simulink model "rlKinovaBallBalance_lags"  (R2024a)
settings: Solver=ode15s  StartTime=0.0  StopTime=inf  MaxStep=0.005  RelTol=1e-4  AbsTol=1e-4
values from neighbouring files (symbols this model uses):
  abs_max_torque_U = [6, 0.70, 2.12, 0.505]    [kinova_params.m]
  g = 3.71    [kinova_params.m]
  max_angular_vel = 2.0    (= 2)    [kinova_params.m]
  max_linear_vel = 0.6    [kinova_params.m]
  max_torque = [1.6; 0.6; 0.9; 0.5]    [kinova_params.m]
  max_torque_PD = [2.5; 0.6; 0.6; 0.3]    [kinova_params.m]
  R1_q0 = 0    [kinova_params.m]
  R2_q0 = deg2rad(20)    [kinova_params.m]
  R3_q0 = 0    [kinova_params.m]
  R4_q0 = deg2rad(135)    [kinova_params.m]
  R5_q0 = 0    [kinova_params.m]
  R6_q0 = deg2rad(-65)    [kinova_params.m]
  R7_q0 = deg2rad(-90)    [kinova_params.m]
  rlEpisodeFinalTime = 21    [kinova_params.m]
  rlStartTime = 0    [kinova_params.m]
  rlTimeStep = 0.01    [kinova_params.m]
  U0 = [-5.75, 0.10, -1.3, 0.0]    [kinova_params.m]
undefined symbols (not defined in the file or in its folder): Control, fluent0, L1, L2, L3, LS1, LS3, plate, R1, R2, R3, Rover, rover_path, RS1, RS3, Ts, vessel, X, Y, Z
libraries: sm_lib x251, nesl_utility x110, fl_lib x85, nesl_utility_internal x34, sdl_lib x20, simulink x16, ee_lib x10, mars_rover_lib x6, slpidlib x2, batteryecm_lib x2, robotalgslib x1, rllib x1
(part 3 of 13)

== system rlKinovaBallBalance_lags/Kinova Ball Balance/7 DOF Manipulator/Shoulder_Link ==
  Actuator1_AxisInvTransform : sm_lib/Frames and Transforms/Rigid Transform  RotationMethod=ArbitraryAxis  FollAlignAxisA=+X  BaseAlignAxisA=+Y  FollAlignAxisB=+Y  BaseAlignAxisB=+Z  RotationStandardAxis=+Z  RotationAngle=0  RotationAngleUnits=rad  RotationArbitraryAxis=[1, 0, 0]  RotationSequenceAxes=FollowerAxes  RotationSequence=XYX  RotationSequenceAngles=[0 0 0]  RotationSequenceAnglesUnits=deg  RotationMatrix=[1 0 0; 0 1 0; 0 0 1]  Quaternion=[1 0 0 0]  TranslationMethod=Cartesian  TranslationCartesianOffset=[0, 0, 0]  TranslationCartesianOffsetUnits=m  TranslationStandardAxis=+Z  TranslationStandardOffset=0  TranslationStandardOffsetUnits=m  TranslationROffset=0  TranslationROffsetUnits=m  TranslationThetaOffset=0  TranslationThetaOffsetUnits=deg  TranslationZOffset=0  TranslationZOffsetUnits=m
  Actuator2_AxisTransform : sm_lib/Frames and Transforms/Rigid Transform  RotationMethod=ArbitraryAxis  FollAlignAxisA=+X  BaseAlignAxisA=+Y  FollAlignAxisB=+Y  BaseAlignAxisB=+Z  RotationStandardAxis=+Z  RotationAngle=0  RotationAngleUnits=rad  RotationArbitraryAxis=[1, 0, 0]  RotationSequenceAxes=FollowerAxes  RotationSequence=XYX  RotationSequenceAngles=[0 0 0]  RotationSequenceAnglesUnits=deg  RotationMatrix=[1 0 0; 0 1 0; 0 0 1]  Quaternion=[1 0 0 0]  TranslationMethod=Cartesian  TranslationCartesianOffset=[0, 0, 0]  TranslationCartesianOffsetUnits=m  TranslationStandardAxis=+Z  TranslationStandardOffset=0  TranslationStandardOffsetUnits=m  TranslationROffset=0  TranslationROffsetUnits=m  TranslationThetaOffset=0  TranslationThetaOffsetUnits=deg  TranslationZOffset=0  TranslationZOffsetUnits=m
  Actuator2_OriginTransform : sm_lib/Frames and Transforms/Rigid Transform  RotationMethod=RotationSequence  FollAlignAxisA=+X  BaseAlignAxisA=+Y  FollAlignAxisB=+Y  BaseAlignAxisB=+Z  RotationStandardAxis=+Z  RotationAngle=0.0  RotationAngleUnits=deg  RotationArbitraryAxis=[0 0 1]  RotationSequenceAxes=BaseAxes  RotationSequence=XYZ  RotationSequenceAngles=[1.5708, 0, 0]  RotationSequenceAnglesUnits=rad  RotationMatrix=[1 0 0; 0 1 0; 0 0 1]  Quaternion=[1 0 0 0]  TranslationMethod=Cartesian  TranslationCartesianOffset=[0, 0.005375, -0.12838]  TranslationCartesianOffsetUnits=m  TranslationStandardAxis=+Z  TranslationStandardOffset=0  TranslationStandardOffsetUnits=m  TranslationROffset=0  TranslationROffsetUnits=m  TranslationThetaOffset=0  TranslationThetaOffsetUnits=deg  TranslationZOffset=0  TranslationZOffsetUnits=m
  Inertia : sm_lib/Body Elements/Inertia  InertiaType=Custom  Mass=2.009  MassUnits=kg  CenterOfMass=[0, 0, 0]  CenterOfMassUnits=m  MomentsOfInertia=[0.004508099999999999, 0.004769500000000001, 0.0013903]  MomentsOfInertiaUnits=kg*m^2  ProductsOfInertia=[-0.00045534, -1.8997e-06, -8.5826e-07]  ProductsOfInertiaUnits=kg*m^2  GraphicType=None  MarkerShape=Inertia  MarkerSize=20  GraphicVisPropType=SimpleVisualProperties  GraphicDiffuseColor=[0.5 0.5 0.5]  GraphicOpacity=1.0  GraphicSpecularColor=[0.5 0.5 0.5 1.0]  GraphicAmbientColor=[0.15 0.15 0.15 1.0]  GraphicEmissiveColor=[0.0 0.0 0.0 1.0]  GraphicShininess=75
  InertiaOriginTransform : sm_lib/Frames and Transforms/Rigid Transform  RotationMethod=RotationSequence  FollAlignAxisA=+X  BaseAlignAxisA=+Y  FollAlignAxisB=+Y  BaseAlignAxisB=+Z  RotationStandardAxis=+Z  RotationAngle=0.0  RotationAngleUnits=deg  RotationArbitraryAxis=[0 0 1]  RotationSequenceAxes=BaseAxes  RotationSequence=XYZ  RotationSequenceAngles=[0, 0, 0]  RotationSequenceAnglesUnits=rad  RotationMatrix=[1 0 0; 0 1 0; 0 0 1]  Quaternion=[1 0 0 0]  TranslationMethod=Cartesian  TranslationCartesianOffset=[-2.2888e-05, -0.010511, -0.075159]  TranslationCartesianOffsetUnits=m  TranslationStandardAxis=+Z  TranslationStandardOffset=0  TranslationStandardOffsetUnits=m  TranslationROffset=0  TranslationROffsetUnits=m  TranslationThetaOffset=0  TranslationThetaOffsetUnits=deg  TranslationZOffset=0  TranslationZOffsetUnits=m
  ReferenceFrame : sm_lib/Frames and Transforms/Reference Frame
  Shoulder Link : Subsystem  Variant=on  VariantControlMode=label  VariantControl=Choice  LabelModeActiveChoice=Choice_1
  VisualOriginTransform : sm_lib/Frames and Transforms/Rigid Transform  RotationMethod=RotationSequence  FollAlignAxisA=+X  BaseAlignAxisA=+Y  FollAlignAxisB=+Y  BaseAlignAxisB=+Z  RotationStandardAxis=+Z  RotationAngle=0.0  RotationAngleUnits=deg  RotationArbitraryAxis=[0 0 1]  RotationSequenceAxes=BaseAxes  RotationSequence=XYZ  RotationSequenceAngles=[0, 0, 0]  RotationSequenceAnglesUnits=rad  RotationMatrix=[1 0 0; 0 1 0; 0 0 1]  Quaternion=[1 0 0 0]  TranslationMethod=Cartesian  TranslationCartesianOffset=[0, 0, 0]  TranslationCartesianOffsetUnits=m  TranslationStandardAxis=+Z  TranslationStandardOffset=0  TranslationStandardOffsetUnits=m  TranslationROffset=0  TranslationROffsetUnits=m  TranslationThetaOffset=0  TranslationThetaOffsetUnits=deg  TranslationZOffset=0  TranslationZOffsetUnits=m
  F : PMIOPort  Side=Left
  F1 : PMIOPort  Port=2  Side=Right
  connections:
  Actuator1_AxisInvTransform/RConn1 -- F/RConn1
  Actuator2_AxisTransform/RConn1 -- F1/RConn1
  Actuator2_AxisTransform/LConn1 -- Actuator2_OriginTransform/RConn1
  Inertia/RConn1 -- InertiaOriginTransform/RConn1
  Actuator2_OriginTransform/LConn1 -- Actuator1_AxisInvTransform/LConn1 -- InertiaOriginTransform/LConn1 -- VisualOriginTransform/LConn1 -- ReferenceFrame/RConn1
  VisualOriginTransform/RConn1 -- Shoulder Link/RConn1

== system rlKinovaBallBalance_lags/Kinova Ball Balance/7 DOF Manipulator/Torque controller J2 ==
  q0 : Inport
  rl_t : Inport  Port=2
  Add Constant : Bias  Bias=U0(1)  SaturateOnIntegerOverflow=off
  Clock : Clock
  Compare To Constant : simulink/Logic and Bit Operations/Compare To Constant  relop=>=  const=rlStartTime  OutDataTypeStr=boolean
  Hold controller J2 : Subsystem
  Saturation : Saturate  UpperLimit=max_torque_PD(1)  LowerLimit=-max_torque_PD(1)
  Simulink-PS Converter1 : nesl_utility_internal/Simulink-PS Converter  PhysicalDomain=network_engine_domain  SubClassName=ps_input  LeftPortType=input  RightPortType=output  PseudoPeriodic=off  Frequencies=[]  NoiseDistribution=none  NoiseParameters=[]  Unit=1  AffineConversion=off  FilteringAndDerivatives=provide  SimscapeFilterOrder=1  InputFilterTimeConstant=0.001  UdotUserProvided=0
  Switch : Switch  Criteria=u2 > Threshold  ZeroCross=off  SaturateOnIntegerOverflow=off  InputSameDT=off
  Transfer Fcn : TransferFcn  Denominator=[0.01 1]
  q : PMIOPort  Side=Right
  w : PMIOPort  Port=2  Side=Right
  output : PMIOPort  Port=3  Side=Right
  torque J2 : Outport
  delta torque J2 : Outport  Port=2
  wires:
  rl_t/1 -> Switch/1
  Compare To Constant/1 -> Switch/2
  q0/1 -> Hold controller J2/1(q0)
  Clock/1 -> Compare To Constant/1
  Switch/1 -> Transfer Fcn/1
  Saturation/1 -> Add Constant/1
  Transfer Fcn/1 -> Simulink-PS Converter1/1
  Hold controller J2/1(hold t) -> delta torque J2/1, Saturation/1
  Add Constant/1 -> torque J2/1, Switch/3
  connections:
  Hold controller J2/LConn1 -- q/RConn1
  Hold controller J2/LConn2 -- w/RConn1
  output/RConn1 -- Simulink-PS Converter1/RConn1

== system rlKinovaBallBalance_lags/Kinova Ball Balance/7 DOF Manipulator/Torque controller J3 ==
  q0 : Inport
  rl_t : Inport  Port=2
  Add Constant : Bias  Bias=U0(2)  SaturateOnIntegerOverflow=off
  Clock : Clock
  Compare To Constant : simulink/Logic and Bit Operations/Compare To Constant  relop=>=  const=rlStartTime  OutDataTypeStr=boolean
  Hold controller J3 : Subsystem
  Saturation : Saturate  UpperLimit=max_torque_PD(2)  LowerLimit=-max_torque_PD(2)
  Simulink-PS Converter1 : nesl_utility_internal/Simulink-PS Converter  PhysicalDomain=network_engine_domain  SubClassName=ps_input  LeftPortType=input  RightPortType=output  PseudoPeriodic=off  Frequencies=[]  NoiseDistribution=none  NoiseParameters=[]  Unit=1  AffineConversion=off  FilteringAndDerivatives=provide  SimscapeFilterOrder=1  InputFilterTimeConstant=0.001  UdotUserProvided=0
  Switch : Switch  Criteria=u2 > Threshold  ZeroCross=off  SaturateOnIntegerOverflow=off  InputSameDT=off
  Transfer Fcn : TransferFcn  Denominator=[0.01 1]
  w : PMIOPort  Side=Right
  q : PMIOPort  Port=2  Side=Right
  output : PMIOPort  Port=3  Side=Right
  delta torque J3 : Outport
  torque J2 : Outport  Port=2
  wires:
  Hold controller J3/1(hold t) -> delta torque J3/1, Saturation/1
  Clock/1 -> Compare To Constant/1
  Switch/1 -> Transfer Fcn/1
  Compare To Constant/1 -> Switch/2
  q0/1 -> Hold controller J3/1(q0)
  Saturation/1 -> Add Constant/1
  rl_t/1 -> Switch/1
  Transfer Fcn/1 -> Simulink-PS Converter1/1
  Add Constant/1 -> Switch/3, torque J2/1
  connections:
  output/RConn1 -- Simulink-PS Converter1/RConn1
  Hold controller J3/LConn2 -- w/RConn1
  Hold controller J3/LConn1 -- q/RConn1

== system rlKinovaBallBalance_lags/Kinova Ball Balance/7 DOF Manipulator/Torque controller J6 ==
  q0 : Inport
  rl_t : Inport  Port=2
  Add Constant : Bias  Bias=U0(3)  SaturateOnIntegerOverflow=off
  Clock : Clock
  Compare To Constant : simulink/Logic and Bit Operations/Compare To Constant  relop=>=  const=rlStartTime  OutDataTypeStr=boolean
  Hold controller J6 : Subsystem
  Saturation : Saturate  UpperLimit=max_torque_PD(3)  LowerLimit=-max_torque_PD(3)
  Simulink-PS Converter1 : nesl_utility_internal/Simulink-PS Converter  PhysicalDomain=network_engine_domain  SubClassName=ps_input  LeftPortType=input  RightPortType=output  PseudoPeriodic=off  Frequencies=[]  NoiseDistribution=none  NoiseParameters=[]  Unit=1  AffineConversion=off  FilteringAndDerivatives=provide  SimscapeFilterOrder=1  InputFilterTimeConstant=0.001  UdotUserProvided=0
  Switch : Switch  Criteria=u2 > Threshold  ZeroCross=off  SaturateOnIntegerOverflow=off  InputSameDT=off
  Transfer Fcn : TransferFcn  Denominator=[0.01 1]
  q : PMIOPort  Side=Right
  output : PMIOPort  Port=2  Side=Right
  w : PMIOPort  Port=3  Side=Right
  delta torque J6 : Outport
  torque J6 : Outport  Port=2
  wires:
  Hold controller J6/1(hold t) -> delta torque J6/1, Saturation/1
  Clock/1 -> Compare To Constant/1
  Switch/1 -> Transfer Fcn/1
  Compare To Constant/1 -> Switch/2
  q0/1 -> Hold controller J6/1(q0)
  Saturation/1 -> Add Constant/1
  rl_t/1 -> Switch/1
  Transfer Fcn/1 -> Simulink-PS Converter1/1
  Add Constant/1 -> Switch/3, torque J6/1
  connections:
  output/RConn1 -- Simulink-PS Converter1/RConn1
  Hold controller J6/LConn2 -- w/RConn1
  Hold controller J6/LConn1 -- q/RConn1

== system rlKinovaBallBalance_lags/Kinova Ball Balance/7 DOF Manipulator/Torque controller J7 ==
  q0 : Inport
  rl_t : Inport  Port=2
  Add Constant : Bias  Bias=U0(4)  SaturateOnIntegerOverflow=off
  Clock : Clock
  Compare To Constant : simulink/Logic and Bit Operations/Compare To Constant  relop=>=  const=rlStartTime  OutDataTypeStr=boolean
  Hold controller J7 : Subsystem
  Saturation : Saturate  UpperLimit=max_torque_PD(4)  LowerLimit=-max_torque_PD(4)
  Simulink-PS Converter1 : nesl_utility_internal/Simulink-PS Converter  PhysicalDomain=network_engine_domain  SubClassName=ps_input  LeftPortType=input  RightPortType=output  PseudoPeriodic=off  Frequencies=[]  NoiseDistribution=none  NoiseParameters=[]  Unit=1  AffineConversion=off  FilteringAndDerivatives=provide  SimscapeFilterOrder=1  InputFilterTimeConstant=0.001  UdotUserProvided=0
  Switch : Switch  Criteria=u2 > Threshold  ZeroCross=off  SaturateOnIntegerOverflow=off  InputSameDT=off
  Transfer Fcn : TransferFcn  Denominator=[0.01 1]
  q : PMIOPort  Side=Right
  w : PMIOPort  Port=2  Side=Right
  output : PMIOPort  Port=3  Side=Right
  delta torque J7 : Outport
  torque J7 : Outport  Port=2
  wires:
  Hold controller J7/1(hold t) -> delta torque J7/1, Saturation/1
  Clock/1 -> Compare To Constant/1
  Compare To Constant/1 -> Switch/2
  q0/1 -> Hold controller J7/1(q0)
  Transfer Fcn/1 -> Simulink-PS Converter1/1
  Switch/1 -> Transfer Fcn/1
  rl_t/1 -> Switch/1
  Saturation/1 -> Add Constant/1
  Add Constant/1 -> torque J7/1, Switch/3
  connections:
  Hold controller J7/LConn2 -- w/RConn1
  Hold controller J7/LConn1 -- q/RConn1
  output/RConn1 -- Simulink-PS Converter1/RConn1

== system rlKinovaBallBalance_lags/Kinova Ball Balance/7 DOF Manipulator/Wrist1_Link ==
  Actuator5_AxisInvTransform : sm_lib/Frames and Transforms/Rigid Transform  RotationMethod=ArbitraryAxis  FollAlignAxisA=+X  BaseAlignAxisA=+Y  FollAlignAxisB=+Y  BaseAlignAxisB=+Z  RotationStandardAxis=+Z  RotationAngle=0  RotationAngleUnits=rad  RotationArbitraryAxis=[1, 0, 0]  RotationSequenceAxes=FollowerAxes  RotationSequence=XYX  RotationSequenceAngles=[0 0 0]  RotationSequenceAnglesUnits=deg  RotationMatrix=[1 0 0; 0 1 0; 0 0 1]  Quaternion=[1 0 0 0]  TranslationMethod=Cartesian  TranslationCartesianOffset=[0, 0, 0]  TranslationCartesianOffsetUnits=m  TranslationStandardAxis=+Z  TranslationStandardOffset=0  TranslationStandardOffsetUnits=m  TranslationROffset=0  TranslationROffsetUnits=m  TranslationThetaOffset=0  TranslationThetaOffsetUnits=deg  TranslationZOffset=0  TranslationZOffsetUnits=m
  Actuator6_AxisTransform : sm_lib/Frames and Transforms/Rigid Transform  RotationMethod=ArbitraryAxis  FollAlignAxisA=+X  BaseAlignAxisA=+Y  FollAlignAxisB=+Y  BaseAlignAxisB=+Z  RotationStandardAxis=+Z  RotationAngle=0  RotationAngleUnits=rad  RotationArbitraryAxis=[1, 0, 0]  RotationSequenceAxes=FollowerAxes  RotationSequence=XYX  RotationSequenceAngles=[0 0 0]  RotationSequenceAnglesUnits=deg  RotationMatrix=[1 0 0; 0 1 0; 0 0 1]  Quaternion=[1 0 0 0]  TranslationMethod=Cartesian  TranslationCartesianOffset=[0, 0, 0]  TranslationCartesianOffsetUnits=m  TranslationStandardAxis=+Z  TranslationStandardOffset=0  TranslationStandardOffsetUnits=m  TranslationROffset=0  TranslationROffsetUnits=m  TranslationThetaOffset=0  TranslationThetaOffsetUnits=deg  TranslationZOffset=0  TranslationZOffsetUnits=m
  Actuator6_OriginTransform : sm_lib/Frames and Transforms/Rigid Transform  RotationMethod=RotationSequence  FollAlignAxisA=+X  BaseAlignAxisA=+Y  FollAlignAxisB=+Y  BaseAlignAxisB=+Z  RotationStandardAxis=+Z  RotationAngle=0.0  RotationAngleUnits=deg  RotationArbitraryAxis=[0 0 1]  RotationSequenceAxes=BaseAxes  RotationSequence=XYZ  RotationSequenceAngles=[1.5708, 0, 0]  RotationSequenceAnglesUnits=rad  RotationMatrix=[1 0 0; 0 1 0; 0 0 1]  Quaternion=[1 0 0 0]  TranslationMethod=Cartesian  TranslationCartesianOffset=[0, 0.00017505, -0.10593]  TranslationCartesianOffsetUnits=m  TranslationStandardAxis=+Z  TranslationStandardOffset=0  TranslationStandardOffsetUnits=m  TranslationROffset=0  TranslationROffsetUnits=m  TranslationThetaOffset=0  TranslationThetaOffsetUnits=deg  TranslationZOffset=0  TranslationZOffsetUnits=m
  Inertia : sm_lib/Body Elements/Inertia  InertiaType=Custom  Mass=0.654  MassUnits=kg  CenterOfMass=[0, 0, 0]  CenterOfMassUnits=m  MomentsOfInertia=[0.0013311, 0.0013282, 0.00030696]  MomentsOfInertiaUnits=kg*m^2  ProductsOfInertia=[-0.00022936, -4.267800000000005e-10, -4.584900000000001e-10]  ProductsOfInertiaUnits=kg*m^2  GraphicType=None  MarkerShape=Inertia  MarkerSize=20  GraphicVisPropType=SimpleVisualProperties  GraphicDiffuseColor=[0.5 0.5 0.5]  GraphicOpacity=1.0  GraphicSpecularColor=[0.5 0.5 0.5 1.0]  GraphicAmbientColor=[0.15 0.15 0.15 1.0]  GraphicEmissiveColor=[0.0 0.0 0.0 1.0]  GraphicShininess=75
  InertiaOriginTransform : sm_lib/Frames and Transforms/Rigid Transform  RotationMethod=RotationSequence  FollAlignAxisA=+X  BaseAlignAxisA=+Y  FollAlignAxisB=+Y  BaseAlignAxisB=+Z  RotationStandardAxis=+Z  RotationAngle=0.0  RotationAngleUnits=deg  RotationArbitraryAxis=[0 0 1]  RotationSequenceAxes=BaseAxes  RotationSequence=XYZ  RotationSequenceAngles=[0, 0, 0]  RotationSequenceAnglesUnits=rad  RotationMatrix=[1 0 0; 0 1 0; 0 0 1]  Quaternion=[1 0 0 0]  TranslationMethod=Cartesian  TranslationCartesianOffset=[-3.2964e-07, -0.009617000000000001, -0.062968]  TranslationCartesianOffsetUnits=m  TranslationStandardAxis=+Z  TranslationStandardOffset=0  TranslationStandardOffsetUnits=m  TranslationROffset=0  TranslationROffsetUnits=m  TranslationThetaOffset=0  TranslationThetaOffsetUnits=deg  TranslationZOffset=0  TranslationZOffsetUnits=m
  ReferenceFrame : sm_lib/Frames and Transforms/Reference Frame
  VisualOriginTransform : sm_lib/Frames and Transforms/Rigid Transform  RotationMethod=RotationSequence  FollAlignAxisA=+X  BaseAlignAxisA=+Y  FollAlignAxisB=+Y  BaseAlignAxisB=+Z  RotationStandardAxis=+Z  RotationAngle=0.0  RotationAngleUnits=deg  RotationArbitraryAxis=[0 0 1]  RotationSequenceAxes=BaseAxes  RotationSequence=XYZ  RotationSequenceAngles=[0, 0, 0]  RotationSequenceAnglesUnits=rad  RotationMatrix=[1 0 0; 0 1 0; 0 0 1]  Quaternion=[1 0 0 0]  TranslationMethod=Cartesian  TranslationCartesianOffset=[0, 0, 0]  TranslationCartesianOffsetUnits=m  TranslationStandardAxis=+Z  TranslationStandardOffset=0  TranslationStandardOffsetUnits=m  TranslationROffset=0  TranslationROffsetUnits=m  TranslationThetaOffset=0  TranslationThetaOffsetUnits=deg  TranslationZOffset=0  TranslationZOffsetUnits=m
  Wrist1 Link : Subsystem  Variant=on  VariantControlMode=label  VariantControl=Choice  LabelModeActiveChoice=Choice_1
  F : PMIOPort  Side=Left
  F1 : PMIOPort  Port=2  Side=Right
  connections:
  Actuator5_AxisInvTransform/RConn1 -- F/RConn1
  Actuator6_AxisTransform/RConn1 -- F1/RConn1
  Actuator6_AxisTransform/LConn1 -- Actuator6_OriginTransform/RConn1
  Inertia/RConn1 -- InertiaOriginTransform/RConn1
  Actuator6_OriginTransform/LConn1 -- Actuator5_AxisInvTransform/LConn1 -- InertiaOriginTransform/LConn1 -- VisualOriginTransform/LConn1 -- ReferenceFrame/RConn1
  VisualOriginTransform/RConn1 -- Wrist1 Link/RConn1

== system rlKinovaBallBalance_lags/Kinova Ball Balance/7 DOF Manipulator/Wrist2_Link ==
  Actuator6_AxisInvTransform : sm_lib/Frames and Transforms/Rigid Transform  RotationMethod=ArbitraryAxis  FollAlignAxisA=+X  BaseAlignAxisA=+Y  FollAlignAxisB=+Y  BaseAlignAxisB=+Z  RotationStandardAxis=+Z  RotationAngle=0  RotationAngleUnits=rad  RotationArbitraryAxis=[1, 0, 0]  RotationSequenceAxes=FollowerAxes  RotationSequence=XYX  RotationSequenceAngles=[0 0 0]  RotationSequenceAnglesUnits=deg  RotationMatrix=[1 0 0; 0 1 0; 0 0 1]  Quaternion=[1 0 0 0]  TranslationMethod=Cartesian  TranslationCartesianOffset=[0, 0, 0]  TranslationCartesianOffsetUnits=m  TranslationStandardAxis=+Z  TranslationStandardOffset=0  TranslationStandardOffsetUnits=m  TranslationROffset=0  TranslationROffsetUnits=m  TranslationThetaOffset=0  TranslationThetaOffsetUnits=deg  TranslationZOffset=0  TranslationZOffsetUnits=m
  Actuator7_AxisTransform : sm_lib/Frames and Transforms/Rigid Transform  RotationMethod=ArbitraryAxis  FollAlignAxisA=+X  BaseAlignAxisA=+Y  FollAlignAxisB=+Y  BaseAlignAxisB=+Z  RotationStandardAxis=+Z  RotationAngle=0  RotationAngleUnits=rad  RotationArbitraryAxis=[1, 0, 0]  RotationSequenceAxes=FollowerAxes  RotationSequence=XYX  RotationSequenceAngles=[0 0 0]  RotationSequenceAnglesUnits=deg  RotationMatrix=[1 0 0; 0 1 0; 0 0 1]  Quaternion=[1 0 0 0]  TranslationMethod=Cartesian  TranslationCartesianOffset=[0, 0, 0]  TranslationCartesianOffsetUnits=m  TranslationStandardAxis=+Z  TranslationStandardOffset=0  TranslationStandardOffsetUnits=m  TranslationROffset=0  TranslationROffsetUnits=m  TranslationThetaOffset=0  TranslationThetaOffsetUnits=deg  TranslationZOffset=0  TranslationZOffsetUnits=m
  Actuator7_OriginTransform : sm_lib/Frames and Transforms/Rigid Transform  RotationMethod=RotationSequence  FollAlignAxisA=+X  BaseAlignAxisA=+Y  FollAlignAxisB=+Y  BaseAlignAxisB=+Z  RotationStandardAxis=+Z  RotationAngle=0.0  RotationAngleUnits=deg  RotationArbitraryAxis=[0 0 1]  RotationSequenceAxes=BaseAxes  RotationSequence=XYZ  RotationSequenceAngles=[-1.5708, 0, 0]  RotationSequenceAnglesUnits=rad  RotationMatrix=[1 0 0; 0 1 0; 0 0 1]  Quaternion=[1 0 0 0]  TranslationMethod=Cartesian  TranslationCartesianOffset=[0, -0.10593, -0.00017505]  TranslationCartesianOffsetUnits=m  TranslationStandardAxis=+Z  TranslationStandardOffset=0  TranslationStandardOffsetUnits=m  TranslationROffset=0  TranslationROffsetUnits=m  TranslationThetaOffset=0  TranslationThetaOffsetUnits=deg  TranslationZOffset=0  TranslationZOffsetUnits=m
  Inertia : sm_lib/Body Elements/Inertia  InertiaType=Custom  Mass=0.654  MassUnits=kg  CenterOfMass=[0, 0, 0]  CenterOfMassUnits=m  MomentsOfInertia=[0.0013422, 0.00031025, 0.001336]  MomentsOfInertiaUnits=kg*m^2  ProductsOfInertia=[0.00023506, -7.338199999999999e-10, 4.959600000000004e-10]  ProductsOfInertiaUnits=kg*m^2  GraphicType=None  MarkerShape=Inertia  MarkerSize=20  GraphicVisPropType=SimpleVisualProperties  GraphicDiffuseColor=[0.5 0.5 0.5]  GraphicOpacity=1.0  GraphicSpecularColor=[0.5 0.5 0.5 1.0]  GraphicAmbientColor=[0.15 0.15 0.15 1.0]  GraphicEmissiveColor=[0.0 0.0 0.0 1.0]  GraphicShininess=75
  InertiaOriginTransform : sm_lib/Frames and Transforms/Rigid Transform  RotationMethod=RotationSequence  FollAlignAxisA=+X  BaseAlignAxisA=+Y  FollAlignAxisB=+Y  BaseAlignAxisB=+Z  RotationStandardAxis=+Z  RotationAngle=0.0  RotationAngleUnits=deg  RotationArbitraryAxis=[0 0 1]  RotationSequenceAxes=BaseAxes  RotationSequence=XYZ  RotationSequenceAngles=[0, 0, 0]  RotationSequenceAnglesUnits=rad  RotationMatrix=[1 0 0; 0 1 0; 0 0 1]  Quaternion=[1 0 0 0]  TranslationMethod=Cartesian  TranslationCartesianOffset=[-3.4377e-07, -0.044043, -0.0097804]  TranslationCartesianOffsetUnits=m  TranslationStandardAxis=+Z  TranslationStandardOffset=0  TranslationStandardOffsetUnits=m  TranslationROffset=0  TranslationROffsetUnits=m  TranslationThetaOffset=0  TranslationThetaOffsetUnits=deg  TranslationZOffset=0  TranslationZOffsetUnits=m
  ReferenceFrame : sm_lib/Frames and Transforms/Reference Frame
  VisualOriginTransform : sm_lib/Frames and Transforms/Rigid Transform  RotationMethod=RotationSequence  FollAlignAxisA=+X  BaseAlignAxisA=+Y  FollAlignAxisB=+Y  BaseAlignAxisB=+Z  RotationStandardAxis=+Z  RotationAngle=0.0  RotationAngleUnits=deg  RotationArbitraryAxis=[0 0 1]  RotationSequenceAxes=BaseAxes  RotationSequence=XYZ  RotationSequenceAngles=[0, 0, 0]  RotationSequenceAnglesUnits=rad  RotationMatrix=[1 0 0; 0 1 0; 0 0 1]  Quaternion=[1 0 0 0]  TranslationMethod=Cartesian  TranslationCartesianOffset=[0, 0, 0]  TranslationCartesianOffsetUnits=m  TranslationStandardAxis=+Z  TranslationStandardOffset=0  TranslationStandardOffsetUnits=m  TranslationROffset=0  TranslationROffsetUnits=m  TranslationThetaOffset=0  TranslationThetaOffsetUnits=deg  TranslationZOffset=0  TranslationZOffsetUnits=m
  Wrist2 Link : Subsystem  Variant=on  VariantControlMode=label  VariantControl=Choice  LabelModeActiveChoice=Choice_1
  F : PMIOPort  Side=Left
  F1 : PMIOPort  Port=2  Side=Right
  connections:
  Actuator6_AxisInvTransform/RConn1 -- F/RConn1
  Actuator7_AxisTransform/RConn1 -- F1/RConn1
  Actuator7_AxisTransform/LConn1 -- Actuator7_OriginTransform/RConn1
  Inertia/RConn1 -- InertiaOriginTransform/RConn1
  Actuator7_OriginTransform/LConn1 -- Actuator6_AxisInvTransform/LConn1 -- InertiaOriginTransform/LConn1 -- VisualOriginTransform/LConn1 -- ReferenceFrame/RConn1
  VisualOriginTransform/RConn1 -- Wrist2 Link/RConn1

== system rlKinovaBallBalance_lags/Kinova Ball Balance/7 DOF Manipulator/base_link ==
  Actuator1_AxisTransform : sm_lib/Frames and Transforms/Rigid Transform  RotationMethod=ArbitraryAxis  FollAlignAxisA=+X  BaseAlignAxisA=+Y  FollAlignAxisB=+Y  BaseAlignAxisB=+Z  RotationStandardAxis=+Z  RotationAngle=0  RotationAngleUnits=rad  RotationArbitraryAxis=[1, 0, 0]  RotationSequenceAxes=FollowerAxes  RotationSequence=XYX  RotationSequenceAngles=[0 0 0]  RotationSequenceAnglesUnits=deg  RotationMatrix=[1 0 0; 0 1 0; 0 0 1]  Quaternion=[1 0 0 0]  TranslationMethod=Cartesian  TranslationCartesianOffset=[0, 0, 0]  TranslationCartesianOffsetUnits=m  TranslationStandardAxis=+Z  TranslationStandardOffset=0  TranslationStandardOffsetUnits=m  TranslationROffset=0  TranslationROffsetUnits=m  TranslationThetaOffset=0  TranslationThetaOffsetUnits=deg  TranslationZOffset=0  TranslationZOffsetUnits=m
  Actuator1_OriginTransform : sm_lib/Frames and Transforms/Rigid Transform  RotationMethod=RotationSequence  FollAlignAxisA=+X  BaseAlignAxisA=+Y  FollAlignAxisB=+Y  BaseAlignAxisB=+Z  RotationStandardAxis=+Z  RotationAngle=0.0  RotationAngleUnits=deg  RotationArbitraryAxis=[0 0 1]  RotationSequenceAxes=BaseAxes  RotationSequence=XYZ  RotationSequenceAngles=[-3.141585307179587, 0, 0]  RotationSequenceAnglesUnits=rad  RotationMatrix=[1 0 0; 0 1 0; 0 0 1]  Quaternion=[1 0 0 0]  TranslationMethod=Cartesian  TranslationCartesianOffset=[0, 0, 0.15643]  TranslationCartesianOffsetUnits=m  TranslationStandardAxis=+Z  TranslationStandardOffset=0  TranslationStandardOffsetUnits=m  TranslationROffset=0  TranslationROffsetUnits=m  TranslationThetaOffset=0  TranslationThetaOffsetUnits=deg  TranslationZOffset=0  TranslationZOffsetUnits=m
  Base Link : Subsystem  Variant=on  VariantControlMode=label  VariantControl=Choice  LabelModeActiveChoice=Choice_1
  ReferenceFrame : sm_lib/Frames and Transforms/Reference Frame
  F : PMIOPort  Side=Left
  F1 : PMIOPort  Port=2  Side=Right
  connections:
  Actuator1_AxisTransform/RConn1 -- F1/RConn1
  Actuator1_AxisTransform/LConn1 -- Actuator1_OriginTransform/RConn1
  F/RConn1 -- Actuator1_OriginTransform/LConn1 -- ReferenceFrame/RConn1 -- Base Link/RConn1

== system rlKinovaBallBalance_lags/Kinova Ball Balance/7 DOF Manipulator/mount ==
  Cylindrical Solid : sm_lib/Body Elements/Cylindrical Solid  CylinderRadius=0.1  CylinderRadiusUnits=m  CylinderLength=0.01  CylinderLengthUnits=m  ExportEntireGeometry=off  InertiaType=CalculateFromGeometry  BasedOnType=Density  Density=1000  DensityUnits=kg/m^3  Mass=1  MassUnits=kg  CenterOfMass=[0 0 0]  CenterOfMassUnits=m  MomentsOfInertia=[1 1 1]  MomentsOfInertiaUnits=kg*m^2  ProductsOfInertia=[0 0 0]  ProductsOfInertiaUnits=kg*m^2  GraphicType=FromGeometry  MarkerShape=Sphere  MarkerSize=10  GraphicVisPropType=SimpleVisualProperties  GraphicDiffuseColor=[0.6 0.6 0.6]  GraphicOpacity=1.0  GraphicSpecularColor=[0.5 0.5 0.5 1.0]  GraphicAmbientColor=[0.15 0.15 0.15 1.0]  GraphicEmissiveColor=[0.0 0.0 0.0 1.0]  GraphicShininess=75  DoExposeReferenceFrame=off  SerializedFrames=<Frames><Frame><Id>Frame1</Id><Value><Name>F1</Name><Origin><Source>GeometricFeature</Source><FeatureName>top surface</FeatureName></Origin><PrimaryAxis><DefinedDirection>+Z</DefinedDirection><Source>ReferenceFrame</Source><SourceDirection>+Z</SourceDirection><FeatureName></FeatureName></PrimaryAxis><SecondaryAxis><DefinedDirection>+X</DefinedDirection><Source>ReferenceFrame</Source><SourceDirection>+X</SourceDirection><FeatureName></FeatureName></SecondaryAxis></Value></Frame><Frame><Id>Frame2</Id><Value><Name>F2</Name><Origin><Source>GeometricFeature</Source><FeatureName>bottom surface</FeatureName></Origin><PrimaryAxis><DefinedDirection>+Z</DefinedDirection><Source>ReferenceFrame</Source><SourceDirection>+Z</SourceDirection><FeatureName></FeatureName></PrimaryAxis><SecondaryAxis><DefinedDirection>+X</DefinedDirection><Source>ReferenceFrame</Source><SourceDirection>+X</SourceDirection><FeatureName></FeatureName></SecondaryAxis></Value></Frame></Frames>
  F : PMIOPort  Side=Right
  F1 : PMIOPort  Port=2  Side=Left
  connections:
  Cylindrical Solid/LConn1 -- F1/RConn1
  F/RConn1 -- Cylindrical Solid/RConn1

== system rlKinovaBallBalance_lags/Kinova Ball Balance/Control/Chassis Control ==
  Waypoints : Inport
  In Bus Element1 : Inport  Port=2  PortName=Chassis  Element=Wheels.Drive
  In Bus Element : Inport  Port=2  PortName=Chassis  Element=Wheels.Steer
  In Bus Element3 : Inport  Port=3  PortName=Body  Element=Pose
  In Bus Element4 : Inport  Port=3  PortName=Body  Element=v
  Ackerman Steer Angle : Subsystem
  Bus Creator : BusCreator  Inputs=3
  Chassis Velocity To Wheel Speed : MATLAB Function  TreatAsAtomicUnit=on
  Constant : Constant  Value=0
  Constant1 : Constant  Value=0
  Constant12 : Constant  Value=Rover.Chassis.Length/2
  Constant2 : Constant  Value=30*pi/180
  Constant8 : Constant  Value=Rover.Wheel.Radius
  Mux2 : Mux  Inputs=6
  Steering Controller : Subsystem  mask{Kp=Control.Steer.Kp, Ki=Control.Steer.Ki, Kd=Control.Steer.Kd, N=Control.Steer.N, Ts_Targetq=Control.Steer.FiltTargetq, Ts_Measq=Control.Steer.FiltSensorq, trq_max_pos=Control.Steer.TrqCmdLimitPos, trq_max_neg=Control.Steer.TrqCmdLimitNeg}
      mask prompts: Kp "Propotional Gain"; Ki "Integral Gain"; Kd "Derivative Gain"; N "Filter Constant (derivative)"; Ts_Targetq "Target Angle (deg)"; Ts_Measq "Sensed Angle (deg)"; trq_max_pos "Torque Command Upper Limit (N*m)"; trq_max_neg "Torque Command Lower Limit (N*m)"
      mask DialogControl cont_pid Prompt: PID Controller
      mask DialogControl cont_filt_ts Prompt: Filter Time Constants
      mask DialogControl cont_trqCmdLim Prompt: Limits at Wheel
  Target Dir To Bicycle Steer Angle : Subsystem  mask{L=1, ld=0.75}
      mask prompts: L "Bicycle length"; ld "Lookahead distance"
      mask TypeOptions L: Bicycle length/Value
      mask TypeOptions ld: Lookahead distance/Value
  Target Direction and Speed : Subsystem
  Vec to Bus SteerTrq : Subsystem
  Vec to Bus qSteer : Subsystem
  Vec to Bus trq : Subsystem
  Vec to Bus wWhl : Subsystem
  Wheel Speed Controller : Subsystem  mask{Kp=Control.Drive.Kp, Ki=Control.Drive.Ki, Kd=Control.Drive.Kd, N=Control.Drive.N, Ts_Targetw=Control.Drive.FiltTargetw, Ts_Measw=Control.Drive.FiltSensorw, trq_max_pos=Control.Drive.TrqCmdLimitPos, trq_max_neg=Control.Drive.TrqCmdLimitNeg}
      mask prompts: Kp "Propotional Gain"; Ki "Integral Gain"; Kd "Derivative Gain"; N "Filter Constant (derivative)"; Ts_Targetw "Target Speed (sec)"; Ts_Measw "Sensed Speed (sec)"; trq_max_pos "Torque Command Upper Limit (N*m)"; trq_max_neg "Torque Command Lower Limit (N*m)"
      mask DialogControl Container4 Prompt: PID Controller
      mask DialogControl cont_filt_ts Prompt: Filter Time Constants
      mask DialogControl cont_trqCmdLim Prompt: Limits
  Bus Element Out1 : Outport  PortName=Ctrl  Element=Steer.trq
  Bus Element Out : Outport  PortName=Ctrl  Element=Drive.trq
  Out Bus Element : Outport  PortName=Ctrl  Element=Cmd.v
  Out Bus Element1 : Outport  PortName=Ctrl  Element=Cmd.qSteer
  Out Bus Element2 : Outport  PortName=Ctrl  Element=Cmd.wWhl
  Out Bus Element3 : Outport  PortName=Ctrl  Element=Camera
  wires:
  Chassis Velocity To Wheel Speed/6(wR3) -> Mux2/6
  Mux2/1 -> Wheel Speed Controller/3(wTarget), Vec to Bus wWhl/1(V)
  Ackerman Steer Angle/4(R3ROC) -> Chassis Velocity To Wheel Speed/5(R3_ROC)
  Chassis Velocity To Wheel Speed/5(wR2) -> Mux2/5
  Chassis Velocity To Wheel Speed/4(wR1) -> Mux2/4
  Ackerman Steer Angle/1(AckSteerAngs) -> Steering Controller/2(qSteerWhl), Vec to Bus qSteer/1(V), Chassis Velocity To Wheel Speed/2(steer_ang)
  Chassis Velocity To Wheel Speed/3(wL3) -> Mux2/3
  Constant12/1 -> Chassis Velocity To Wheel Speed/7(L)
  Constant8/1 -> Chassis Velocity To Wheel Speed/6(wheel_r)
  Chassis Velocity To Wheel Speed/2(wL2) -> Mux2/2
  Chassis Velocity To Wheel Speed/1(wL1) -> Mux2/1
  Ackerman Steer Angle/3(L3ROC) -> Chassis Velocity To Wheel Speed/4(L3_ROC)
  Ackerman Steer Angle/2(A3 ROC) -> Chassis Velocity To Wheel Speed/3(A3_ROC)
  Target Dir To Bicycle Steer Angle/1(qSteer) -> Ackerman Steer Angle/2(Delta)
  Wheel Speed Controller/1(trq) -> Vec to Bus trq/1(V)
  Steering Controller/1(trq) -> Vec to Bus SteerTrq/1(V)
  Vec to Bus trq/1(B) -> Bus Element Out/1
  Vec to Bus SteerTrq/1(B) -> Bus Element Out1/1
  In Bus Element1/1 -> Wheel Speed Controller/1(Meas)
  In Bus Element/1 -> Steering Controller/1(Meas)
  Vec to Bus qSteer/1(B) -> Out Bus Element1/1
  Vec to Bus wWhl/1(B) -> Out Bus Element2/1
  Target Direction and Speed/1(StopAtGoal) -> Wheel Speed Controller/2(StopAtGoal), Steering Controller/3(RoverAtGoal)
  Target Direction and Speed/2(vTarget) -> Chassis Velocity To Wheel Speed/1(vTarget), Out Bus Element/1
  In Bus Element3/1 -> Target Direction and Speed/2(Pose)
  Waypoints/1 -> Target Direction and Speed/3(WP)
  Target Direction and Speed/3(AtGoal) -> Ackerman Steer Angle/1(AtGoal)
  Target Direction and Speed/4(TargetDir) -> Target Dir To Bicycle Steer Angle/1(TargetDir)
  In Bus Element4/1 -> Target Direction and Speed/1(vRover)
  Constant/1 -> Bus Creator/1  "mp"
  Constant1/1 -> Bus Creator/2  "my"
  Constant2/1 -> Bus Creator/3  "hp"
  Bus Creator/1 -> Out Bus Element3/1

== system rlKinovaBallBalance_lags/Kinova Ball Balance/Observation/a_GVM_prev-10 ==
  a_GVM : Inport
  Unit Delay{,1..9} (10 alike) : UnitDelay  SampleTime=-1  HasFrameUpgradeWarning=on
  Out1 : Outport
  wires:
  Unit Delay4/1 -> Unit Delay8/1
  Unit Delay1/1 -> Unit Delay2/1
  Unit Delay/1 -> Unit Delay1/1
  Unit Delay3/1 -> Unit Delay9/1
  Unit Delay9/1 -> Unit Delay7/1
  Unit Delay5/1 -> Unit Delay4/1
  Unit Delay7/1 -> Unit Delay6/1
  Unit Delay8/1 -> Out1/1
  Unit Delay6/1 -> Unit Delay5/1
  Unit Delay2/1 -> Unit Delay3/1
  a_GVM/1 -> Unit Delay/1

== system rlKinovaBallBalance_lags/Kinova Ball Balance/Observation/act_torque_prev-10 ==
  In1 : Inport
  Unit Delay{,1..9} (10 alike) : UnitDelay  SampleTime=-1  HasFrameUpgradeWarning=on
  Out1 : Outport
  wires:
  Unit Delay4/1 -> Unit Delay8/1
  Unit Delay1/1 -> Unit Delay2/1
  Unit Delay/1 -> Unit Delay1/1
  Unit Delay3/1 -> Unit Delay9/1
  Unit Delay9/1 -> Unit Delay7/1
  Unit Delay5/1 -> Unit Delay4/1
  Unit Delay7/1 -> Unit Delay6/1
  Unit Delay8/1 -> Out1/1
  Unit Delay6/1 -> Unit Delay5/1
  Unit Delay2/1 -> Unit Delay3/1
  In1/1 -> Unit Delay/1

== system rlKinovaBallBalance_lags/Kinova Ball Balance/Observation/com_GVM_loc_prev-1 ==
  com_GVM_loc : Inport
  Unit Delay{,1..9} (10 alike) : UnitDelay  SampleTime=-1  HasFrameUpgradeWarning=on
  Out1 : Outport
  wires:
  Unit Delay4/1 -> Unit Delay8/1
  Unit Delay1/1 -> Unit Delay2/1
  Unit Delay/1 -> Unit Delay1/1
  Unit Delay3/1 -> Unit Delay9/1
  Unit Delay9/1 -> Unit Delay7/1
  Unit Delay5/1 -> Unit Delay4/1
  Unit Delay7/1 -> Unit Delay6/1
  Unit Delay8/1 -> Out1/1
  Unit Delay6/1 -> Unit Delay5/1
  Unit Delay2/1 -> Unit Delay3/1
  com_GVM_loc/1 -> Unit Delay/1

== system rlKinovaBallBalance_lags/Kinova Ball Balance/Observation/com_GVM_loc_prev-10 ==
  com_GVM_loc : Inport
  Unit Delay{,1..9} (10 alike) : UnitDelay  SampleTime=-1  HasFrameUpgradeWarning=on
  Out1 : Outport
  wires:
  Unit Delay4/1 -> Unit Delay8/1
  Unit Delay1/1 -> Unit Delay2/1
  Unit Delay/1 -> Unit Delay1/1
  Unit Delay3/1 -> Unit Delay9/1
  Unit Delay9/1 -> Unit Delay7/1
  Unit Delay5/1 -> Unit Delay4/1
  Unit Delay7/1 -> Unit Delay6/1
  Unit Delay8/1 -> Out1/1
  Unit Delay6/1 -> Unit Delay5/1
  Unit Delay2/1 -> Unit Delay3/1
  com_GVM_loc/1 -> Unit Delay/1

== system rlKinovaBallBalance_lags/Kinova Ball Balance/Observation/com_GVM_loc_prev-20 ==
  com_GVM_loc : Inport
  Lag 10-1 : Subsystem
  Lag 10-2 : Subsystem
  Out1 : Outport
  wires:
  com_GVM_loc/1 -> Lag 10-1/1(In1)
  Lag 10-1/1(Out1) -> Lag 10-2/1(In1)
  Lag 10-2/1(Out1) -> Out1/1

== system rlKinovaBallBalance_lags/Kinova Ball Balance/Observation/m_liquid_prev-10 ==
  In1 : Inport
  Unit Delay{,1..9} (10 alike) : UnitDelay  SampleTime=-1  HasFrameUpgradeWarning=on
  Out1 : Outport
  wires:
  Unit Delay4/1 -> Unit Delay8/1
  Unit Delay1/1 -> Unit Delay2/1
  Unit Delay/1 -> Unit Delay1/1
  Unit Delay3/1 -> Unit Delay9/1
  Unit Delay9/1 -> Unit Delay7/1
  Unit Delay5/1 -> Unit Delay4/1
  Unit Delay7/1 -> Unit Delay6/1
  Unit Delay8/1 -> Out1/1
  Unit Delay6/1 -> Unit Delay5/1
  Unit Delay2/1 -> Unit Delay3/1
  In1/1 -> Unit Delay/1

== system rlKinovaBallBalance_lags/Kinova Ball Balance/Observation/m_liquid_prev-20 ==
  In1 : Inport
  Lag 1 : Subsystem
  Lag 10 : Subsystem
  Out1 : Outport
  wires:
  In1/1 -> Lag 10/1(In1)
  Lag 10/1(Out1) -> Lag 1/1(In1)
  Lag 1/1(Out1) -> Out1/1
